simulink model "bess_frequency_scan"  (R2024b)
settings: Solver=ode23t  StartTime=0.0  StopTime=simulation_stop_time_s  RelTol=1e-3
InitFcn:
  | init_phase1;
undefined symbols (not defined in the file): battery_capacity_Ah, battery_initial_soc_pu, case_step_time_s, Cf_F, command_delay_samples, ctrl_sample_time_s, current_noise_variance, dcdc_gate_sample_time_s, DiscIntNeverNeededParam, L1_H, L2_H, P_recovery_W, P_ref_final_W, P_ref_initial_W, Q_recovery_var, Q_ref_final_var, Q_ref_initial_var, R1_Ohm, R2_Ohm, Rd_Ohm, recovery_time_s, soc_max_pu, soc_min_pu, Vdc_ref_final_V, Vdc_ref_initial_V, voltage_noise_variance
libraries: nesl_utility x11, ee_lib x10, fl_lib x5, batteryecm_lib x1
settings Model: Creator=Legion  LastModifiedBy=Legion

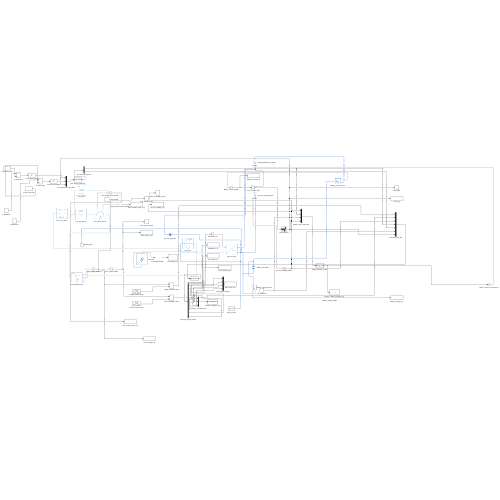
[thumbnail: Simulink's stored preview of the top-level diagram]
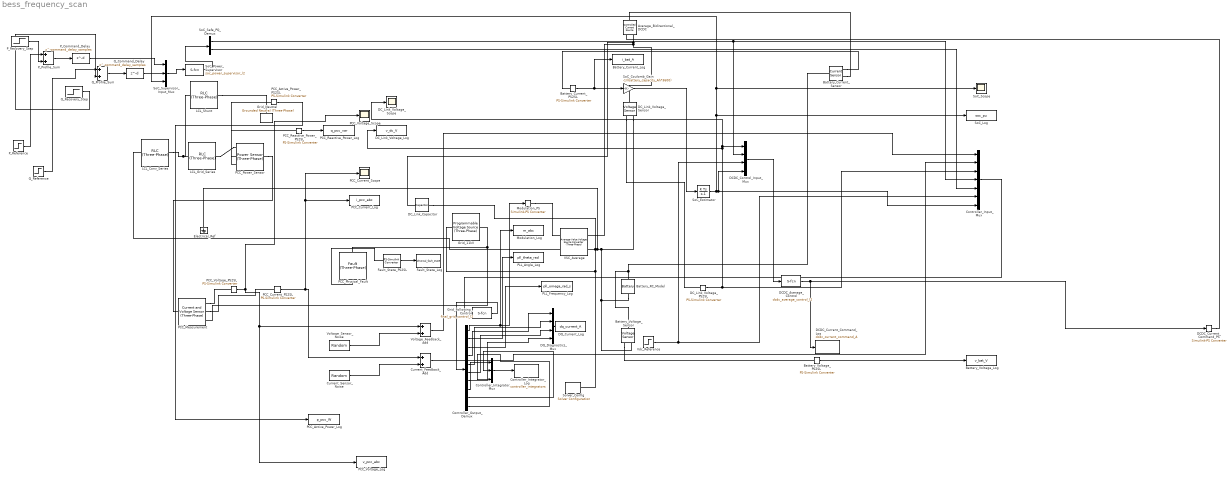
== system bess_frequency_scan ==
  Average_Bidirectional_DCDC : fl_lib/Electrical/Electrical Sources/Controlled Current Source
  Battery_Current_Log : ToWorkspace  VariableName=i_bat_A  SaveFormat=Timeseries  SampleTime=-1
  Battery_Current_PS2SL : nesl_utility/PS-Simulink Converter  PhysicalDomain=network_engine_domain  SubClassName=ps_output  LeftPortType=input  RightPortType=output  PseudoPeriodic=off  Frequencies=[]  VectorFormat=inherit  Unit=inherit  AffineConversion=off
  Battery_Current_Sensor : fl_lib/Electrical/Electrical Sensors/Current Sensor
  Battery_RC_Model : batteryecm_lib/Battery  Vnom=battery_nominal_voltage_V V  prm_dir=simscape.enum.battery.prm_dir.disabled  R1_dis=2 Ohm  R1_ch=2 Ohm  R1=battery_series_resistance_Ohm Ohm  prm_AH=simscape.enum.battery.prm_AH.finite  AH=battery_capacity_Ah A*hr  V1=battery_voltage_at_half_charge_V V  AH1=25 A*hr  prm_R2=simscape.enum.battery.prm_R2.disabled  R2=2000 Ohm  Tmeas=298.15 K  charge_measurement_port=simscape.enum.battery.enable.no  prm_dyn=simscape.enum.battery.prm_dyn.rc1  Rp1=battery_rc_resistance_Ohm Ohm  tau1=battery_rc_time_constant_s s  Rp2=0.005 Ohm  tau2=30 s  Rp3=0.005 Ohm  tau3=30 s  Rp4=0.005 Ohm  tau4=30 s  Rp5=0.005 Ohm  tau5=30 s  prm_fade=simscape.enum.battery.prm_fade.disabled  N_fade=100  AH_fade=45 A*hr  R1_fade=2.02 Ohm  R1_ch_fade=2.02 Ohm  V1_fade=10.35 V  prm_age=simscape.enum.battery.prm_age.disabled  prm_age_OCV=simscape.enum.battery.prm_age_OCV.OCV  OCV_age=0.9  SOC_age=60  Tmeas_age=298.15 K  delta_time_age_vec=[0] d  temperature_age_vec=[273] K  OCV_scaling_age=2.2134e6  OCV_offset_age=1.632e6  temp_exp_age=0.515833569 V  t_exp_age=0.75  Vnom_T2=12 V  R1_T2=2.2 Ohm  R1_T2_dis=2.2 Ohm  R1_T2_ch=2.2 Ohm  V1_T2=11.4 V  R2_T2=2200 Ohm  Rp1_T2=0.005 Ohm  tau1_T2=30 s  Rp2_T2=0.005 Ohm  tau2_T2=30 s  Rp3_T2=0.005 Ohm  tau3_T2=30 s  Rp4_T2=0.005 Ohm  tau4_T2=30 s  Rp5_T2=0.005 Ohm  tau5_T2=30 s  Tmeas2=273.15 K  thermal_port=simscape.enum.thermaleffects.omit  thermal_mass=30000 J/K  i_specify=off  i_priority=None  i=0 A  i_nominal_specify=off  i_nominal_value=1  i_nominal_unit=A  v_specify=off  v_priority=None  v=0 V  v_nominal_specify=off  v_nominal_value=1  v_nominal_unit=V  charge_specify=on  charge_priority=High  charge=battery_initial_charge_Ah A*hr  charge_nominal_specify=off  charge_nominal_value=1  charge_nominal_unit=A*hr  num_cycles_specify=off  num_cycles_priority=High  num_cycles=0  num_cycles_nominal_specify=off  num_cycles_nominal_value=1  num_cycles_nominal_unit=1  temperature_specify=off  temperature_priority=High  temperature=298.15 K  temperature_nominal_specify=off  temperature_nominal_value=1  temperature_nominal_unit=K
      settings: LibrarySourceBlock=batt_lib/Cells/Battery
  Battery_Voltage_Log : ToWorkspace  VariableName=v_bat_V  SaveFormat=Timeseries  SampleTime=-1
  Battery_Voltage_PS2SL : nesl_utility/PS-Simulink Converter  PhysicalDomain=network_engine_domain  SubClassName=ps_output  LeftPortType=input  RightPortType=output  PseudoPeriodic=off  Frequencies=[]  VectorFormat=inherit  Unit=inherit  AffineConversion=off
  Battery_Voltage_Sensor : fl_lib/Electrical/Electrical Sensors/Voltage Sensor
  Controller_Input_Mux : Mux  Inputs=7
  Controller_Integrator_Log : ToWorkspace  VariableName=controller_integrators  SaveFormat=Structure With Time  SampleTime=-1
  Controller_Integrator_Mux : Mux  Inputs=3
  Controller_Output_Demux : Demux  Outputs=[3 1 1 1 1 1 1 1 1 1]
  Current_Feedback_Add : Sum
  Current_Sensor_Noise : RandomNumber  Mean=[0 0 0]  Variance=current_noise_variance  Seed=[201 202 203]  SampleTime=ctrl_sample_time_s
  DCDC_Average_Control : M-S-Function  FunctionName=dcdc_average_control_l2  Parameters=dcdc_cfg
  DCDC_Control_Input_Mux : Mux
  DCDC_Current_Command_Log : ToWorkspace  VariableName=dcdc_current_command_A  SaveFormat=Structure With Time  SampleTime=-1
  DCDC_Current_Command_PS : nesl_utility/Simulink-PS Converter  PhysicalDomain=network_engine_domain  SubClassName=ps_input  LeftPortType=input  RightPortType=output  PseudoPeriodic=off  Frequencies=[]  NoiseDistribution=none  NoiseParameters=[]  Unit=1  AffineConversion=off  FilteringAndDerivatives=provide  SimscapeFilterOrder=1  InputFilterTimeConstant=0.001  UdotUserProvided=0
  DC_Link_Capacitor : ee_lib/Passive/Capacitor  cap_option=ee.enum.passive.capacitor.capOption.const  c=dclink_capacitance_F F  Cvec=[1e-05, 1e-06] F  Vvec=[0, 10] V  CV_table_symmetry=ee.enum.passive.capacitor.tableSymmetry.yes  f_vec=[1, 10] kHz  DFext_vec=[.8, 1.2]  enable_C_tol=ee.enum.toleranceApplication.none  averaging_period=0 s  C_tol=5  tol_distribution=ee.enum.toleranceDistribution.uniform  nSigma=4  r=0 Ohm  g=0 1/Ohm  enable_operating_limits=ee.enum.enable.no  operating_limit_action=ee.enum.passive.reportOpLim.warn  max_working_voltage_range=[-25, 25] V  power_rating=1 W  maxTemperature=85 degC  thermalEnable=false  thermalMass=1 J/K  fault_action=simscape.enum.assert.action.none  t_fault=1 s  i_specify=off  i_priority=None  i=0 A  i_nominal_specify=off  i_nominal_value=1  i_nominal_unit=A  v_specify=on  v_priority=High  v=Vdc_test_V V  v_nominal_specify=off  v_nominal_value=1  v_nominal_unit=V  vc_specify=on  vc_priority=High  vc=Vdc_test_V V  vc_nominal_specify=off  vc_nominal_value=1  vc_nominal_unit=V  T_specify=off  T_priority=None  T=298.15 K  T_nominal_specify=off  T_nominal_value=1  T_nominal_unit=K
  DC_Link_Voltage_Log : ToWorkspace  VariableName=v_dc_V  SaveFormat=Timeseries  SampleTime=-1
  DC_Link_Voltage_PS2SL : nesl_utility/PS-Simulink Converter  PhysicalDomain=network_engine_domain  SubClassName=ps_output  LeftPortType=input  RightPortType=output  PseudoPeriodic=off  Frequencies=[]  VectorFormat=inherit  Unit=inherit  AffineConversion=off
  DC_Link_Voltage_Scope : Scope
  DC_Link_Voltage_Sensor : fl_lib/Electrical/Electrical Sensors/Voltage Sensor
  DQ_Current_Log : ToWorkspace  VariableName=dq_current_A  SaveFormat=Timeseries  SampleTime=-1
  DQ_Diagnostics_Mux : Mux
  Electrical_Ref : fl_lib/Electrical/Electrical Elements/Electrical Reference
  Fault_State_Log : ToWorkspace  VariableName=physical_fault_state  SaveFormat=Timeseries  SampleTime=-1
  Fault_State_PS2SL : nesl_utility/PS-Simulink Converter  PhysicalDomain=network_engine_domain  SubClassName=ps_output  LeftPortType=input  RightPortType=output  PseudoPeriodic=off  Frequencies=[]  VectorFormat=inherit  Unit=inherit  AffineConversion=off
  Grid_11kV : ee_lib/Sources/Programmable Voltage Source (Three-Phase)  magnitude_type=ee.enum.timechanging.constant  vline_rms=V_grid_LL_rms_V V  magn_ramp=1 V/s  magn_step=1 V  magn_modu_magn=1 V  magn_modu_freq=1 Hz  magn_t1=1 s  magn_t2=2 s  frequency_type=ee.enum.timechanging.constant  freq=f_grid_Hz Hz  freq_ramp=1 Hz/s  freq_step=1 Hz  freq_modu_magn=1 Hz  freq_modu_freq=1 Hz  freq_t1=1 s  freq_t2=2 s  phase_type=ee.enum.timechanging.constant  shift=0 deg  phase_ramp=1 deg/s  phase_step=1 deg  phase_modu_magn=1 deg  phase_modu_freq=1 Hz  phase_t1=1 s  phase_t2=2 s  impedance_option=1  SShortCircuit=S_sc_grid_VA A*V  XR=X_R_grid  R=0.01 Ohm  L=3.97e-4 H  G_parasitic=1e-6 1/Ohm  harmonic_option=0  harmonic_orders=[5, 7, 11, 13]  harmonic_ratios=[.1, .1, .1, .1]  harmonic_shifts=[0, 0, 0, 0] deg  harmonic_sequences=[1, 1, 1, 1]  harmonic_t1=-inf s  harmonic_t2=inf s  I_specify=off  I_priority=None  I=[0, 0, 0] A  I_nominal_specify=off  I_nominal_value=1  I_nominal_unit=A  V_specify=off  V_priority=None  V=[0, 0, 0] V  V_nominal_specify=off  V_nominal_value=1  V_nominal_unit=V
      settings: InternalSimscapePortConfiguration="{\"Bottom\":[],\"Left\":[{\"id\":\"n\",\"label\":\"n\",\"type\":\"foundation.electrical.electrical\"}],\"Right\":[{\"id\":\"N\",\"label\":\"~\",\"type\":\"foundation.electrical.three_phase\"}],\"Top\":[]}"
  Grid_Following_Control : M-S-Function  FunctionName=final_grid_control_l2  Parameters=ctrl_cfg
  Grid_Neutral : ee_lib/Connectors & References/Grounded Neutral (Three-Phase)
  LCL_Conv_Series : ee_lib/Passive/RLC Assemblies/RLC (Three-Phase)  port_option=ee.enum.threePhasePort.composite  component_structure=ee.enum.rlc.structure.SeriesRL  R=R1_Ohm Ohm  L=L1_H H  C=1e-6 F  R_parasitic=0 Ohm  G_parasitic=0 1/Ohm  IL_specify=off  IL_priority=High  IL=[0, 0, 0] A  IL_nominal_specify=off  IL_nominal_value=1  IL_nominal_unit=A  VC_specify=off  VC_priority=High  VC=[0, 0, 0] V  VC_nominal_specify=off  VC_nominal_value=1  VC_nominal_unit=V
      settings: InternalSimscapePortConfiguration="{\"Bottom\":[],\"Left\":[{\"id\":\"N1\",\"label\":\"~1\",\"type\":\"foundation.electrical.three_phase\"}],\"Right\":[{\"id\":\"N2\",\"label\":\"~2\",\"type\":\"foundation.electrical.three_phase\"}],\"Top\":[]}"
  LCL_Grid_Series : ee_lib/Passive/RLC Assemblies/RLC (Three-Phase)  port_option=ee.enum.threePhasePort.composite  component_structure=ee.enum.rlc.structure.SeriesRL  R=R2_Ohm Ohm  L=L2_H H  C=1e-6 F  R_parasitic=0 Ohm  G_parasitic=0 1/Ohm  IL_specify=off  IL_priority=High  IL=[0, 0, 0] A  IL_nominal_specify=off  IL_nominal_value=1  IL_nominal_unit=A  VC_specify=off  VC_priority=High  VC=[0, 0, 0] V  VC_nominal_specify=off  VC_nominal_value=1  VC_nominal_unit=V
      settings: InternalSimscapePortConfiguration="{\"Bottom\":[],\"Left\":[{\"id\":\"N1\",\"label\":\"~1\",\"type\":\"foundation.electrical.three_phase\"}],\"Right\":[{\"id\":\"N2\",\"label\":\"~2\",\"type\":\"foundation.electrical.three_phase\"}],\"Top\":[]}"
  LCL_Shunt : ee_lib/Passive/RLC Assemblies/RLC (Three-Phase)  port_option=ee.enum.threePhasePort.composite  component_structure=ee.enum.rlc.structure.SeriesRC  R=Rd_Ohm Ohm  L=1e-3 H  C=Cf_F F  R_parasitic=0 Ohm  G_parasitic=0 1/Ohm  IL_specify=off  IL_priority=High  IL=[0, 0, 0] A  IL_nominal_specify=off  IL_nominal_value=1  IL_nominal_unit=A  VC_specify=off  VC_priority=High  VC=[0, 0, 0] V  VC_nominal_specify=off  VC_nominal_value=1  VC_nominal_unit=V
      settings: InternalSimscapePortConfiguration="{\"Bottom\":[],\"Left\":[{\"id\":\"N1\",\"label\":\"~1\",\"type\":\"foundation.electrical.three_phase\"}],\"Right\":[{\"id\":\"N2\",\"label\":\"~2\",\"type\":\"foundation.electrical.three_phase\"}],\"Top\":[]}"
  Modulation_Log : ToWorkspace  VariableName=m_abc  SaveFormat=Timeseries  SampleTime=-1
  Modulation_PS : nesl_utility/Simulink-PS Converter  PhysicalDomain=network_engine_domain  SubClassName=ps_input  LeftPortType=input  RightPortType=output  PseudoPeriodic=off  Frequencies=[]  NoiseDistribution=none  NoiseParameters=[]  Unit=1  AffineConversion=off  FilteringAndDerivatives=provide  SimscapeFilterOrder=1  InputFilterTimeConstant=0.001  UdotUserProvided=0
  PCC_Active_Power_Log : ToWorkspace  VariableName=p_pcc_W  SaveFormat=Timeseries  SampleTime=-1
  PCC_Active_Power_PS2SL : nesl_utility/PS-Simulink Converter  PhysicalDomain=network_engine_domain  SubClassName=ps_output  LeftPortType=input  RightPortType=output  PseudoPeriodic=off  Frequencies=[]  VectorFormat=inherit  Unit=W  AffineConversion=off
  PCC_Current_Log : ToWorkspace  VariableName=i_pcc_abc  SaveFormat=Timeseries  SampleTime=-1
  PCC_Current_PS2SL : nesl_utility/PS-Simulink Converter  PhysicalDomain=network_engine_domain  SubClassName=ps_output  LeftPortType=input  RightPortType=output  PseudoPeriodic=off  Frequencies=[]  VectorFormat=1-D array  Unit=A  AffineConversion=off
  PCC_Current_Scope : Scope
  PCC_Measurement : ee_lib/Sensors & Transducers/Current and Voltage Sensor (Three-Phase)  vMeasurementType=ee.enum.vmeasurement.ll  outputUnit=ee.enum.unit.si  SRated=P_rated_W A*V  VRated=V_grid_LL_rms_V V  I_specify=off  I_priority=None  I=[0, 0, 0] A  I_nominal_specify=off  I_nominal_value=1  I_nominal_unit=A  V_specify=off  V_priority=None  V=[0, 0, 0] V  V_nominal_specify=off  V_nominal_value=1  V_nominal_unit=V
      settings: InternalSimscapePortConfiguration="{\"Bottom\":[],\"Left\":[{\"id\":\"N1\",\"label\":\"~1\",\"type\":\"foundation.electrical.three_phase\"}],\"Right\":[{\"id\":\"V_output\",\"label\":\"V\",\"type\":\"output\"},{\"id\":\"I_output\",\"label\":\"I\",\"type\":\"output\"},{\"id\":\"N2\",\"label\":\"~2\",\"type\":\"foundation.electrical.three_phase\"}],\"Top\":[]}"
  PCC_Physical_Fault : ee_lib/Utilities/Fault (Three-Phase)  fault_type_option=0  R_pn_fault=physical_fault_resistance_Ohm Ohm  R_ng_fault=physical_fault_ground_resistance_Ohm Ohm  exposemeasurement=ee.enum.exposemeasurement.visible  enable_external_fault=ee.enum.external_fault.hidden  fault_threshold=0.5  fault_condition=1  fault_resettable=0  enable_temporal_fault=0  fault_start_time=1 s  fault_duration=0.1 s  G_parasitic=1e-6 1/Ohm
      settings: InternalSimscapePortConfiguration="{\"Bottom\":[],\"Left\":[{\"id\":\"N\",\"label\":\"~\",\"type\":\"foundation.electrical.three_phase\"}],\"Right\":[{\"id\":\"X\",\"label\":\"X\",\"type\":\"output\"}],\"Top\":[]}"
  PCC_Power_Sensor : ee_lib/Sensors & Transducers/Power Sensor (Three-Phase)  load_type=ee.enum.passive.type_balanced.balanced  f0=60 Hz  config=ee.enum.with_neutral.no  rho=1
      settings: InternalSimscapePortConfiguration="{\"Bottom\":[],\"Left\":[{\"id\":\"N1\",\"label\":\"~1\",\"type\":\"foundation.electrical.three_phase\"}],\"Right\":[{\"id\":\"N2\",\"label\":\"~2\",\"type\":\"foundation.electrical.three_phase\"}],\"Top\":[{\"id\":\"Pm\",\"label\":\"P\",\"type\":\"output\"},{\"id\":\"Qm\",\"label\":\"Q\",\"type\":\"output\"}]}"
  PCC_Reactive_Power_Log : ToWorkspace  VariableName=q_pcc_var  SaveFormat=Timeseries  SampleTime=-1
  PCC_Reactive_Power_PS2SL : nesl_utility/PS-Simulink Converter  PhysicalDomain=network_engine_domain  SubClassName=ps_output  LeftPortType=input  RightPortType=output  PseudoPeriodic=off  Frequencies=[]  VectorFormat=inherit  Unit=inherit  AffineConversion=off
  PCC_Voltage_Log : ToWorkspace  VariableName=v_pcc_abc  SaveFormat=Timeseries  SampleTime=-1
  PCC_Voltage_PS2SL : nesl_utility/PS-Simulink Converter  PhysicalDomain=network_engine_domain  SubClassName=ps_output  LeftPortType=input  RightPortType=output  PseudoPeriodic=off  Frequencies=[]  VectorFormat=1-D array  Unit=V  AffineConversion=off
  PCC_Voltage_Scope : Scope
  PLL_Angle_Log : ToWorkspace  VariableName=pll_theta_rad  SaveFormat=Timeseries  SampleTime=-1
  PLL_Frequency_Log : ToWorkspace  VariableName=pll_omega_rad_s  SaveFormat=Timeseries  SampleTime=-1
  P_Command_Delay : Delay  DelayLength=command_delay_samples  InitialCondition=P_ref_initial_W  SampleTime=ctrl_sample_time_s
  P_Profile_Sum : Sum
  P_Recovery_Step : Step  Time=recovery_time_s  After=P_recovery_W-P_ref_final_W  SampleTime=ctrl_sample_time_s
  P_Reference : Step  Time=case_step_time_s  Before=P_ref_initial_W  After=P_ref_final_W  SampleTime=ctrl_sample_time_s
  Q_Command_Delay : Delay  DelayLength=command_delay_samples  InitialCondition=Q_ref_initial_var  SampleTime=ctrl_sample_time_s
  Q_Profile_Sum : Sum
  Q_Recovery_Step : Step  Time=recovery_time_s  After=Q_recovery_var-Q_ref_final_var  SampleTime=ctrl_sample_time_s
  Q_Reference : Step  Time=case_step_time_s  Before=Q_ref_initial_var  After=Q_ref_final_var  SampleTime=ctrl_sample_time_s
  SoC_Coulomb_Gain : Gain  Gain=-1/(battery_capacity_Ah*3600)
  SoC_Estimator : DiscreteIntegrator  InitialCondition=battery_initial_soc_pu  SampleTime=dcdc_gate_sample_time_s  LimitOutput=on  UpperSaturationLimit=soc_max_pu  LowerSaturationLimit=soc_min_pu  ICPrevOutput=DiscIntNeverNeededParam  ICPrevScaledInput=DiscIntNeverNeededParam
  SoC_Log : ToWorkspace  VariableName=soc_pu  SaveFormat=Timeseries  SampleTime=-1
  SoC_Power_Supervisor : M-S-Function  FunctionName=soc_power_supervisor_l2  Parameters=soc_supervisor_cfg
  SoC_Safe_PQ_Demux : Demux  Outputs=2
  SoC_Scope : Scope
  SoC_Supervisor_Input_Mux : Mux  Inputs=3
  Solver_Config : nesl_utility/Solver Configuration  PhysicalDomain=network_engine_domain  SubClassName=solver  LeftPortType=input  RightPortType=generic  Tones=[]  Harmonics=[]  SimulateNoise=off  Profile=off  UseLocalSampling=off  EnableSwitchedLinearOptims=on  FrequencyDomain=off  UseCCode=off  RelTol=0.001  AbsTol=0.001  MinStep=1e-09  ToWorkspace=off  RevertToSquareIcSolve=off  NumHomotopyIterations=100  PhasorMode=off  PhasorModeNumHarmonics=1  ConsistencySolver=NEWTON_XTOL_AFTER_FTOL  IndexReductionMethod=DerivativeReplacement  DoDC=off  ResidualTolerance=1e-09  ConsistencyTolSource=GLOBAL  ConsistencyAbsTol=0.001  ConsistencyRelTol=0.001  ConsistencyTolFactor=0.001  UseLocalSolver=off  LocalSolverChoice=NE_BACKWARD_EULER_ADVANCER  ResolveIndetEquations=on  FunctionEvalNumThread=1  LocalSolverSampleTime=0.001  DoFixedCost=off  MaxNonlinIter=3  MaxModeIter=2  ComputeImpulses=off  ImpulseIterations=2  LinearAlgebra=auto  LinearAlgebraNumThread=0  EquationFormulation=NE_TIME_EF  DelaysMemoryBudget=1024  AutomaticFiltering=on  FilteringTimeConstant=0.001  PartitionStorageMethod=AS_NEEDED  PartitionMemoryBudget=1024  PartitionMethod=ROBUST  MultibodyUseLocalSolver=off  MultibodyLocalSolverChoice=ODE1  MultibodyLocalSolverSampleTime=0.001
  VSC_Average : ee_lib/Semiconductors & Converters/Converters/Average-Value Voltage Source Converter (Three-Phase)  port_option=ee.enum.threePhasePort.composite  frequency_option=ee.enum.converters.frequency.variable  input_option=ee.enum.converters.inputOption.ModWave  FRated=f_grid_Hz Hz  losses_parameterization=ee.enum.converters.losses.fixed  Pfixed=1 W  ks=0.01  kc1=1.7 V  kc2=0.01 Ohm  Ploss_vect=[100, 800, 1870, 3250, 4900] W  Irms_vect=[10, 100, 200, 300, 400] A  Vdc_nom=Vdc_test_V V  thermal_mass=30000 J/K  temperature_specify=off  temperature_priority=High  temperature=298.15 K  temperature_nominal_specify=off  temperature_nominal_value=1  temperature_nominal_unit=K
      settings: InternalSimscapePortConfiguration="{\"Bottom\":[],\"Left\":[{\"id\":\"ModWave\",\"label\":\"ModWave\",\"type\":\"input\"},{\"id\":\"N\",\"label\":\"~\",\"type\":\"foundation.electrical.three_phase\"}],\"Right\":[{\"id\":\"p\",\"label\":\"+\",\"type\":\"foundation.electrical.electrical\"},{\"id\":\"n\",\"label\":\"-\",\"type\":\"foundation.electrical.electrical\"}],\"Top\":[]}"
  Vdc_Reference : Step  Time=case_step_time_s  Before=Vdc_ref_initial_V  After=Vdc_ref_final_V  SampleTime=ctrl_sample_time_s
  Voltage_Feedback_Add : Sum
  Voltage_Sensor_Noise : RandomNumber  Mean=[0 0 0]  Variance=voltage_noise_variance  Seed=[101 102 103]  SampleTime=ctrl_sample_time_s
  wires:
  Q_Recovery_Step/1 -> Q_Profile_Sum/2
  Q_Profile_Sum/1 -> Q_Command_Delay/1
  Q_Reference/1 -> Q_Profile_Sum/1
  P_Profile_Sum/1 -> P_Command_Delay/1
  P_Recovery_Step/1 -> P_Profile_Sum/2
  P_Reference/1 -> P_Profile_Sum/1
  SoC_Safe_PQ_Demux/2 -> Controller_Input_Mux/5
  PCC_Voltage_PS2SL/1 -> PCC_Voltage_Log/1, Voltage_Feedback_Add/1, PCC_Voltage_Scope/1
  PCC_Current_PS2SL/1 -> PCC_Current_Scope/1, PCC_Current_Log/1, Current_Feedback_Add/1
  DC_Link_Voltage_PS2SL/1 -> DC_Link_Voltage_Scope/1, DCDC_Control_Input_Mux/1, DC_Link_Voltage_Log/1, Controller_Input_Mux/3
  SoC_Safe_PQ_Demux/1 -> DCDC_Control_Input_Mux/2, Controller_Input_Mux/4
  SoC_Estimator/1 -> Controller_Input_Mux/7, DCDC_Control_Input_Mux/4, SoC_Supervisor_Input_Mux/3, SoC_Scope/1, SoC_Log/1
  Controller_Input_Mux/1 -> Grid_Following_Control/1
  SoC_Supervisor_Input_Mux/1 -> SoC_Power_Supervisor/1
  Vdc_Reference/1 -> DCDC_Control_Input_Mux/3, Controller_Input_Mux/6
  P_Command_Delay/1 -> SoC_Supervisor_Input_Mux/1
  Q_Command_Delay/1 -> SoC_Supervisor_Input_Mux/2
  Voltage_Feedback_Add/1 -> Controller_Input_Mux/1
  Current_Feedback_Add/1 -> Controller_Input_Mux/2
  Current_Sensor_Noise/1 -> Current_Feedback_Add/2
  Voltage_Sensor_Noise/1 -> Voltage_Feedback_Add/2
  Fault_State_PS2SL/1 -> Fault_State_Log/1
  SoC_Power_Supervisor/1 -> SoC_Safe_PQ_Demux/1
  SoC_Coulomb_Gain/1 -> SoC_Estimator/1
  Battery_Current_PS2SL/1 -> Battery_Current_Log/1, SoC_Coulomb_Gain/1
  Battery_Voltage_PS2SL/1 -> Battery_Voltage_Log/1
  PCC_Active_Power_PS2SL/1 -> PCC_Active_Power_Log/1
  DQ_Diagnostics_Mux/1 -> DQ_Current_Log/1
  PCC_Reactive_Power_PS2SL/1 -> PCC_Reactive_Power_Log/1
  Controller_Integrator_Mux/1 -> Controller_Integrator_Log/1
  Controller_Output_Demux/10 -> Controller_Integrator_Mux/3
  Controller_Output_Demux/9 -> Controller_Integrator_Mux/2
  Controller_Output_Demux/8 -> Controller_Integrator_Mux/1
  Controller_Output_Demux/7 -> DQ_Diagnostics_Mux/4
  Controller_Output_Demux/6 -> DQ_Diagnostics_Mux/3
  Controller_Output_Demux/5 -> DQ_Diagnostics_Mux/2
  Controller_Output_Demux/4 -> DQ_Diagnostics_Mux/1
  Controller_Output_Demux/3 -> PLL_Frequency_Log/1
  Controller_Output_Demux/2 -> PLL_Angle_Log/1
  Controller_Output_Demux/1 -> Modulation_Log/1, Modulation_PS/1
  Grid_Following_Control/1 -> Controller_Output_Demux/1
  DCDC_Control_Input_Mux/1 -> DCDC_Average_Control/1
  DCDC_Average_Control/1 -> DCDC_Current_Command_Log/1, DCDC_Current_Command_PS/1
  connections:
  DC_Link_Voltage_Sensor/LConn1 -- Average_Bidirectional_DCDC/RConn2 -- DC_Link_Capacitor/LConn1 -- VSC_Average/RConn1
  DC_Link_Voltage_Sensor/RConn2 -- Battery_RC_Model/RConn1 -- Battery_Voltage_Sensor/RConn2 -- Grid_11kV/LConn1 -- Solver_Config/RConn1 -- VSC_Average/RConn2 -- DC_Link_Capacitor/RConn1 -- Electrical_Ref/LConn1
  PCC_Physical_Fault/LConn1 -- Grid_11kV/RConn1 -- PCC_Measurement/RConn3
  Battery_Voltage_Sensor/LConn1 -- Battery_RC_Model/LConn1 -- Battery_Current_Sensor/LConn1
  LCL_Grid_Series/LConn1 -- LCL_Conv_Series/RConn1 -- LCL_Shunt/LConn1
  PCC_Power_Sensor/RConn1 -- PCC_Measurement/LConn1
  PCC_Measurement/RConn1 -- PCC_Voltage_PS2SL/LConn1
  PCC_Measurement/RConn2 -- PCC_Current_PS2SL/LConn1
  PCC_Physical_Fault/RConn1 -- Fault_State_PS2SL/LConn1
  Battery_Current_Sensor/RConn1 -- Battery_Current_PS2SL/LConn1
  DC_Link_Voltage_Sensor/RConn1 -- DC_Link_Voltage_PS2SL/LConn1
  DCDC_Current_Command_PS/RConn1 -- Average_Bidirectional_DCDC/RConn1
  Battery_Current_Sensor/RConn2 -- Average_Bidirectional_DCDC/LConn1
  Modulation_PS/RConn1 -- VSC_Average/LConn1
  VSC_Average/LConn2 -- LCL_Conv_Series/LConn1
  Battery_Voltage_Sensor/RConn1 -- Battery_Voltage_PS2SL/LConn1
  LCL_Grid_Series/RConn1 -- PCC_Power_Sensor/LConn1
  PCC_Power_Sensor/LConn2 -- PCC_Active_Power_PS2SL/LConn1
  PCC_Power_Sensor/LConn3 -- PCC_Reactive_Power_PS2SL/LConn1
  LCL_Shunt/RConn1 -- Grid_Neutral/LConn1
